simulink model "disturbanceEffectOn_second_order_closed"  (R2023b)
settings: Solver=VariableStepAuto  StartTime=0.0  StopTime=10.0  RelTol=1e-3
settings Model: Creator=reemb  LastModifiedBy=reemb

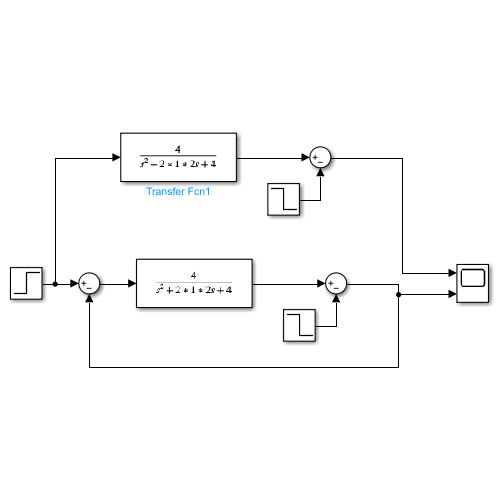
[thumbnail: Simulink's stored preview of the top-level diagram]
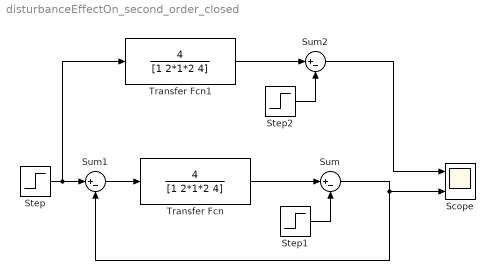
== system disturbanceEffectOn_second_order_closed ==
  Scope : Scope  NumInputPorts=2
  Step : Step  SampleTime=0
  Step1 : Step  Time=5  After=-1.7  SampleTime=0
  Step2 : Step  Time=5  After=-1.7  SampleTime=0
  Sum : Sum  Inputs=|+-
  Sum1 : Sum  Inputs=|+-
  Sum2 : Sum  Inputs=|+-
  Transfer Fcn : TransferFcn  Numerator=[4]  Denominator=[1 2*1*2 4]
  Transfer Fcn1 : TransferFcn  Numerator=[4]  Denominator=[1 2*1*2 4]
  wires:
  Step/1 -> Transfer Fcn1/1, Sum1/1
  Transfer Fcn/1 -> Sum/1
  Sum1/1 -> Transfer Fcn/1
  Sum/1 -> Sum1/2, Scope/2
  Step1/1 -> Sum/2
  Step2/1 -> Sum2/2
  Sum2/1 -> Scope/1
  Transfer Fcn1/1 -> Sum2/1
